simulink model "voima_7"  (R2022a)
settings: Solver=ode15s  StartTime=0.0  StopTime=1000  MaxStep=1  RelTol=1e-3  AbsTol=1e-3
values from neighbouring files (symbols this model uses):
  D = 1.2/a*0.5*tau    (= 37.7655389457)    [ex10.m]    (also in ex3.m = PID(3,i); ex4.m = 0; ex6.m = 37.77; ex7.m)
  fkul_0 = 35.7    [ex10.m]    (also in ex2.m; ex3.m; ex4.m; ex5.m)
  fp_0 = 35.7    [ex10.m]    (also in ex2.m; ex3.m; ex4.m; ex5.m)
  h1 = 8.3    [ex10.m]    (also in ex2.m; ex3.m; ex4.m; ex5.m)
  h2 = 21.0    (= 21)    [ex10.m]    (also in ex2.m; ex3.m; ex4.m; ex5.m)
  I = (1.2/a)/(2*tau)    (= 0.147521636507)    [ex10.m]    (also in ex3.m = PID(2,i); ex6.m = 0.1; ex7.m; ex8.m)
  k0 = 1.0    (= 1)    [ex10.m]    (also in ex2.m; ex3.m; ex4.m; ex5.m)
  k1 = 2.0    (= 2)    [ex10.m]    (also in ex2.m; ex3.m; ex4.m; ex5.m)
  k2 = 1/30    (= 0.0333333333333)    [ex10.m]    (also in ex2.m; ex3.m; ex4.m; ex5.m)
  k3 = 0.4    [ex10.m]    (also in ex2.m; ex3.m; ex4.m; ex5.m)
  k4 = 1/300    (= 0.00333333333333)    [ex10.m]    (also in ex2.m; ex3.m; ex4.m; ex5.m)
  k5 = 0.6    [ex10.m]    (also in ex2.m; ex3.m; ex4.m; ex5.m)
  k6 = 0.6    [ex10.m]    (also in ex2.m; ex3.m; ex4.m; ex5.m)
  k_in = k_in*15    (= 382.5)    [ex10.m]    (also in ex2.m = 25.5; ex3.m = 25.5; ex4.m = 25.5; ex5.m = 25.5)
  k_out = k_out*15    (= 3150)    [ex10.m]    (also in ex2.m = 210; ex3.m = 210; ex4.m = 210; ex5.m = 210)
  ma_0 = 150000.0    (= 150000)    [ex10.m]    (also in ex2.m; ex3.m; ex4.m; ex5.m)
  P = 1.2/a    (= 4.72069236821)    [ex10.m]    (also in ex3.m = PID(1,i); ex6.m = 5.66; ex7.m; ex8.m)
  pa_0 = 10.0    (= 10)    [ex10.m]    (also in ex2.m; ex3.m; ex4.m; ex5.m)
  pcp = 13.0    (= 13)    [ex10.m]    (also in ex2.m; ex3.m; ex4.m; ex5.m)
  pk_0 = 91.0    (= 91)    [ex10.m]    (also in ex2.m; ex3.m; ex4.m; ex5.m)
  pkp_0 = 89.25    [ex10.m]    (also in ex2.m; ex3.m; ex4.m; ex5.m)
  pvp_0 = 3.0    (= 3)    [ex10.m]    (also in ex2.m; ex3.m; ex4.m; ex5.m)
  T1 = 30.0    (= 30)    [ex10.m]    (also in ex2.m; ex3.m; ex4.m; ex5.m)
  Ts = 15.0    (= 15)    [ex10.m]    (also in ex2.m; ex3.m; ex4.m; ex5.m)
libraries: slpidlib x1
settings Model: Creator=meharju1  LastModifiedBy=Chris
settings SolverCC: AutoScaleAbsTol=off  AlgebraicLoopSolver=TrustRegion
settings DataIOCC: SaveFormat=Array  SignalLoggingSaveFormat=ModelDataLogs  SaveOutput=off  TimeSaveName=t
settings OptimizationCC: DefaultParameterBehavior=Inlined  InlineInvariantSignals=on  ExpressionDepthLimit=2147483647  EfficientFloat2IntCast=on  LifeSpan=inf
settings DebuggingCC: SaveWithParameterizedLinksMsg=none  MultiTaskCondExecSysMsg=none  UnconnectedInputMsg=warning  UnconnectedOutputMsg=warning  UnconnectedLineMsg=warning  UniqueDataStoreMsg=error  StateNameClashWarn=warning  PregeneratedLibrarySubsystemCodeDiagnostic=none  StrictBusMsg=ErrorOnBusTreatedAsVector  SFUnexpectedBacktrackingDiag=warning  SFNoUnconditionalDefaultTransitionDiag=warning  SFExecutionAtInitializationDiag=none  SFMachineParentedDataDiag=warning  ArithmeticOperatorsInVariantConditions=warning
settings HardwareCC: ProdBitPerPointer=32  ProdBitPerSizeT=32  ProdBitPerPtrDiffT=32  ProdLargestAtomicFloat=None  ProdIntDivRoundTo=Undefined  ProdEndianess=Unspecified  ProdWordSize=32  ProdHWDeviceType=32-bit Generic  TargetUnknown=on
settings ModelReferenceCC: PropagateSignalLabelsOutOfModel=off
settings SFSimCC: SimUseLocalCustomCode=off  CustomCodeUndefinedFunction=UseInterfaceOnly
settings RTWCC: RTWUseLocalCustomCode=off
settings CodeAppCC: StateflowObjectComments=on
settings GRTTargetCC: TargetLangStandard=C89/C90 (ANSI)  CombineOutputUpdateFcns=off  GRTInterface=on
settings ConfigComp: CovMetricSettings=dw  CovSaveCumulativeToWorkspaceVar=on  CovSaveSingleToWorkspaceVar=on  CovExternalEMLEnable=off

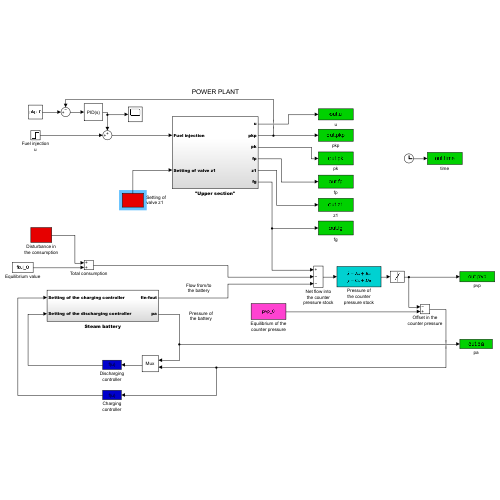
[thumbnail: Simulink's stored preview of the top-level diagram]
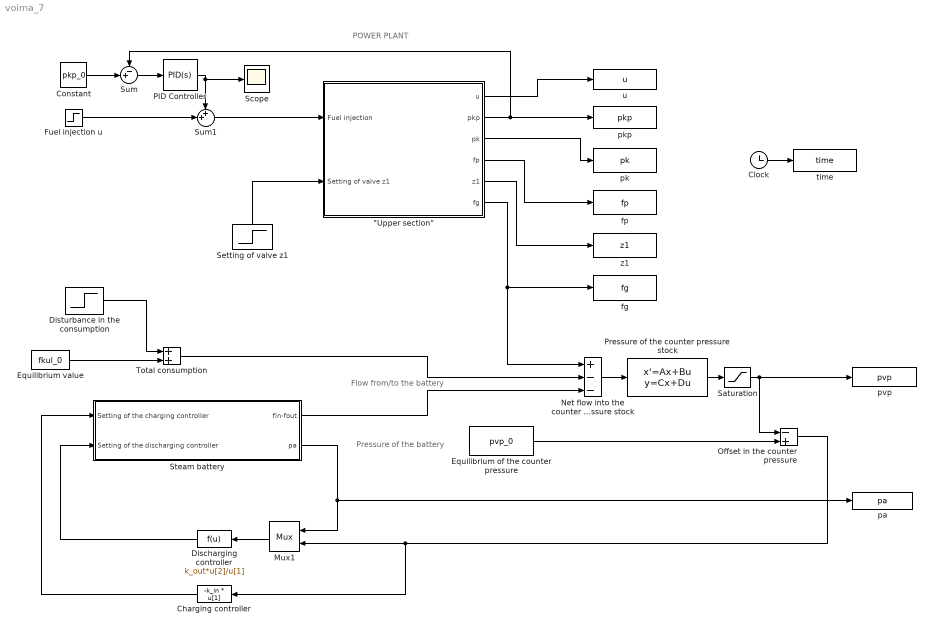
== system voima_7 ==
  note: POWER PLANT
  note: Flow from/to
      | the battery
  note: Pressure of
      | the battery
  "\"Upper section\"" : Subsystem
  Charging controller : Fcn  Expr=-k_in * u[1]
  Clock : Clock
  Constant : Constant  Value=pkp_0
  Discharging controller : Fcn  Expr=k_out*u[2]/u[1]
  Disturbance in the consumption : Step  Time=200  After=2  SampleTime=0
  Equilibrium of the counter pressure : Constant  Value=pvp_0
  Equilibrium value : Constant  Value=fkul_0
  Fuel injection u : Step  Time=200  Before=35.7  After=35.7  SampleTime=0
  Mux1 : Mux  Inputs=2
  Net flow into the counter pressure stock : Sum  Inputs=+--  InputSameDT=on  SaturateOnIntegerOverflow=on  OutDataTypeStr=Inherit: Same as first input
  Offset in the counter pressure : Sum  Inputs=-+  InputSameDT=on  SaturateOnIntegerOverflow=on  OutDataTypeStr=Inherit: Same as first input
  PID Controller : slpidlib/PID Controller  Controller=PID  Form=Parallel  TimeDomain=Continuous-time  UseExternalTs=off  SampleTime=-1  IntegratorMethod=Forward Euler  FilterMethod=Forward Euler  ControllerParametersSource=internal  P=P  I=I  UseKiTs=off  D=D  N=100  UseFilter=on  TunerSelectOption=Transfer Function Based (PID Tuner App)  InitialConditionSource=internal  InitialConditionForIntegrator=0  InitialConditionForFilter=0  DifferentiatorICPrevScaledInput=0  ExternalReset=none  TrackingMode=off  Kt=1  LimitOutput=off  SatLimitsSource=internal  UpperSaturationLimit=inf  LowerSaturationLimit=-inf  LinearizeAsGain=on  AntiWindupMode=none  Kb=1  POutMin=[]  POutMax=[]  IOutMin=[]  IOutMax=[]  DOutMin=[]  DOutMax=[]  NOutMin=[]  NOutMax=[]  SumOutMin=[]  SumOutMax=[]  SaturationOutMin=[]  SaturationOutMax=[]  PParamMin=[]  PParamMax=[]  IParamMin=[]  IParamMax=[]  DParamMin=[]  DParamMax=[]  NParamMin=[]  NParamMax=[]  KbParamMin=[]  KbParamMax=[]  KtParamMin=[]  KtParamMax=[]  KbOutMin=[]  KbOutMax=[]  KtOutMin=[]  KtOutMax=[]  IntegratorOutMin=[]  IntegratorOutMax=[]  FilterOutMin=[]  FilterOutMax=[]  SumI1OutMin=[]  SumI1OutMax=[]  SumI2OutMin=[]  SumI2OutMax=[]  SumI3OutMin=[]  SumI3OutMax=[]  SumI4OutMin=[]  SumI4OutMax=[]  SumDOutMin=[]  SumDOutMax=[]  DifferentiatorOutMin=[]  DifferentiatorOutMax=[]  FilterDiffOutCoefMin=[]  FilterDiffOutCoefMax=[]  ReciprocalOutMin=[]  ReciprocalOutMax=[]  SumDenOutMin=[]  SumDenOutMax=[]  SumNumOutMin=[]  SumNumOutMax=[]  DivideOutMin=[]  DivideOutMax=[]  UdiffTsProdOutMin=[]  UdiffTsProdOutMax=[]  NTsProdOutMin=[]  NTsProdOutMax=[]  UintegralTsProdOutMin=[]  UintegralTsProdOutMax=[]  UngainTsProdOutMin=[]  UngainTsProdOutMax=[]  IntegratorContinuousStateAttributes=''  IntegratorStateMustResolveToSignalObject=off  IntegratorRTWStateStorageClass=Auto  FilterContinuousStateAttributes=''  FilterStateMustResolveToSignalObject=off  FilterRTWStateStorageClass=Auto  ParallelPVariant=InternalParameters  IdealPVariant=Disabled  IVariant=InternalParameters  DVariant=InternalParameters  IntegratorVariant=Continuous  SatVariant=Disabled  AWVariant=Passthrough  PCopyVariant=Disabled  TRVariant=Disabled  FdbkBlocksVariant=Forward  IdealPFdbkVariant=Disabled  SatFdbkVariant=Disabled  DerivativeFilterVariant=ContFilter  NVariant=InternalParameters  NCopyVariant=Disabled  FilterICVariant=InternalICsFilter  IntegratorICVariant=InternalICs  ExternalResetVariant=Disabled  TRSumVariant=Passthrough  SumFdbkVariant=Disabled  SumVariant=Sum_PID  TsampFilterVariant=InternalTs  TsampNgainVariant=Passthrough  TsampIntegralVariant=Passthrough  ExternalSaturationOutDataTypeStr=Inherit: Same as second input  aMode=0
  Pressure of the counter pressure stock : StateSpace  A=0  B=k4  D=0  InitialCondition=pvp_0
  Saturation : Saturate  UpperLimit=100000  LowerLimit=0
  Scope : Scope
  Setting of valve z1 : Step  Time=200  Before=1  SampleTime=0
  Steam battery : Subsystem
  Sum : Sum  Inputs=-+|
  Sum1 : Sum  Inputs=++|
  Total consumption : Sum  InputSameDT=on  SaturateOnIntegerOverflow=on  OutDataTypeStr=Inherit: Same as first input
  fg : ToWorkspace  VariableName=fg
      settings: MaxDataPoints=2000
  fp : ToWorkspace  VariableName=fp
      settings: MaxDataPoints=2000
  pa : ToWorkspace  VariableName=pa
      settings: MaxDataPoints=2000
  pk : ToWorkspace  VariableName=pk
      settings: MaxDataPoints=2000
  pkp : ToWorkspace  VariableName=pkp
      settings: MaxDataPoints=2000
  pvp : ToWorkspace  VariableName=pvp
      settings: MaxDataPoints=2000
  time : ToWorkspace  VariableName=time
      settings: MaxDataPoints=2000
  u : ToWorkspace  VariableName=u
      settings: MaxDataPoints=2000
  z1 : ToWorkspace  VariableName=z1
      settings: MaxDataPoints=2000
  wires:
  Net flow into the counter pressure stock/1 -> Pressure of the counter pressure stock/1
  Equilibrium value/1 -> Total consumption/2
  Disturbance in the consumption/1 -> Total consumption/1
  Mux1/1 -> Discharging controller/1
  Equilibrium of the counter pressure/1 -> Offset in the counter pressure/2
  Steam battery/2(pa) -> pa/1, Mux1/1
  Total consumption/1 -> Net flow into the counter pressure stock/2
  Steam battery/1(fin-fout) -> Net flow into the counter pressure stock/3
  Discharging controller/1 -> Steam battery/2(Setting of the discharging controller)
  Offset in the counter pressure/1 -> Mux1/2, Charging controller/1
  "\"Upper section\""/1(u) -> u/1
  "\"Upper section\""/2(pkp) -> pkp/1, Sum/1
  "\"Upper section\""/3(pk) -> pk/1
  "\"Upper section\""/4(fp) -> fp/1
  Setting of valve z1/1 -> "\"Upper section\""/2(Setting of valve z1)
  Fuel injection u/1 -> Sum1/2
  Pressure of the counter pressure stock/1 -> Saturation/1
  Saturation/1 -> pvp/1, Offset in the counter pressure/1
  "\"Upper section\""/6(fg) -> Net flow into the counter pressure stock/1, fg/1
  "\"Upper section\""/5(z1) -> z1/1
  Charging controller/1 -> Steam battery/1(Setting of the charging controller)
  Clock/1 -> time/1
  Sum/1 -> PID Controller/1
  PID Controller/1 -> Scope/1, Sum1/1
  Constant/1 -> Sum/2
  Sum1/1 -> "\"Upper section\""/1(Fuel injection)

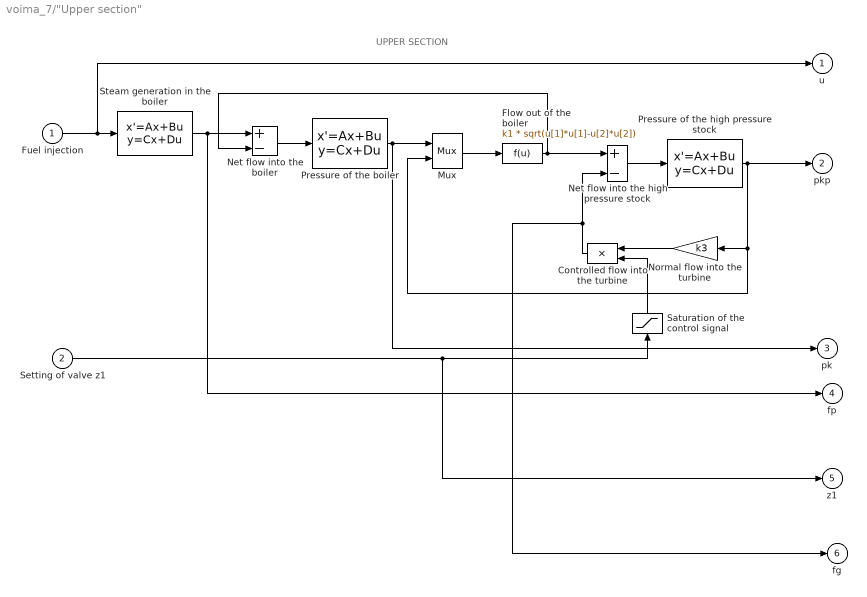
== system voima_7/"Upper section" ==
  note: UPPER SECTION
  Fuel injection : Inport
  Setting of valve z1 : Inport  Port=2
  Controlled flow into the turbine : Product  InputSameDT=on  RndMeth=Zero  SaturateOnIntegerOverflow=on  OutDataTypeStr=Inherit: Same as first input
  Flow out of the boiler : Fcn  Expr=k1 * sqrt(u[1]*u[1]-u[2]*u[2])
  Mux : Mux  Inputs=2
  Net flow into the boiler : Sum  Inputs=+-  InputSameDT=on  SaturateOnIntegerOverflow=on  OutDataTypeStr=Inherit: Same as first input
  Net flow into the high pressure stock : Sum  Inputs=+-  InputSameDT=on  SaturateOnIntegerOverflow=on  OutDataTypeStr=Inherit: Same as first input
  Normal flow into the turbine : Gain  Gain=k3  SaturateOnIntegerOverflow=on  OutDataTypeStr=Inherit: Same as input  ParamDataTypeStr=Inherit: Same as input
  Pressure of the boiler : StateSpace  A=0  B=1/Ts  D=0  InitialCondition=pk_0
  Pressure of the high pressure stock : StateSpace  A=0  B=k2  D=0  InitialCondition=pkp_0
  Saturation of the control signal : Saturate  UpperLimit=1.2  LowerLimit=0.8
  Steam generation in the boiler : StateSpace  A=-1/T1  B=k0 / T1  D=0  InitialCondition=fp_0
  u : Outport  VectorParamsAs1DForOutWhenUnconnected=off
  pkp : Outport  Port=2  VectorParamsAs1DForOutWhenUnconnected=off
  pk : Outport  Port=3  VectorParamsAs1DForOutWhenUnconnected=off
  fp : Outport  Port=4  VectorParamsAs1DForOutWhenUnconnected=off
  z1 : Outport  Port=5  VectorParamsAs1DForOutWhenUnconnected=off
  fg : Outport  Port=6  VectorParamsAs1DForOutWhenUnconnected=off
  wires:
  Saturation of the control signal/1 -> Controlled flow into the turbine/2
  Normal flow into the turbine/1 -> Controlled flow into the turbine/1
  Pressure of the high pressure stock/1 -> Normal flow into the turbine/1, Mux/2, pkp/1
  Net flow into the high pressure stock/1 -> Pressure of the high pressure stock/1
  Flow out of the boiler/1 -> Net flow into the boiler/2, Net flow into the high pressure stock/1
  Mux/1 -> Flow out of the boiler/1
  Net flow into the boiler/1 -> Pressure of the boiler/1
  Pressure of the boiler/1 -> Mux/1, pk/1
  Steam generation in the boiler/1 -> Net flow into the boiler/1, fp/1
  Controlled flow into the turbine/1 -> Net flow into the high pressure stock/2, fg/1
  Fuel injection/1 -> Steam generation in the boiler/1, u/1
  Setting of valve z1/1 -> Saturation of the control signal/1, z1/1

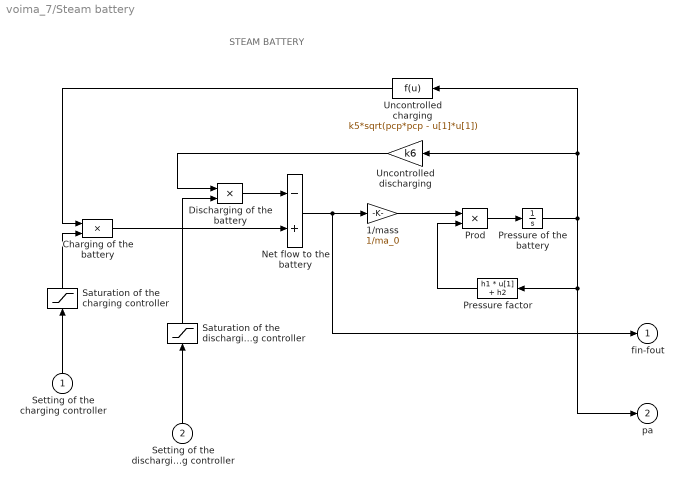
== system voima_7/Steam battery ==
  note: STEAM BATTERY
  Setting of the charging controller : Inport
  Setting of the discharging controller : Inport  Port=2
  1/mass : Gain  Gain=1/ma_0  SaturateOnIntegerOverflow=on  OutDataTypeStr=Inherit: Same as input  ParamDataTypeStr=Inherit: Same as input
  Charging of the battery : Product  InputSameDT=on  RndMeth=Zero  SaturateOnIntegerOverflow=on  OutDataTypeStr=Inherit: Same as first input
  Discharging of the battery : Product  InputSameDT=on  RndMeth=Zero  SaturateOnIntegerOverflow=on  OutDataTypeStr=Inherit: Same as first input
  Net flow to the battery : Sum  Inputs=-+  InputSameDT=on  SaturateOnIntegerOverflow=on  OutDataTypeStr=Inherit: Same as first input
  Pressure factor : Fcn  Expr="h1 * u[1]  + h2"
  Pressure of the battery : Integrator  InitialCondition=pa_0
  Prod : Product  InputSameDT=on  RndMeth=Zero  SaturateOnIntegerOverflow=on  OutDataTypeStr=Inherit: Same as first input
  Saturation of the charging controller : Saturate  UpperLimit=0  LowerLimit=0
  Saturation of the discharging controller : Saturate  UpperLimit=0  LowerLimit=0
  Uncontrolled charging : Fcn  Expr=k5*sqrt(pcp*pcp - u[1]*u[1])
  Uncontrolled discharging : Gain  Gain=k6  SaturateOnIntegerOverflow=on  OutDataTypeStr=Inherit: Same as input  ParamDataTypeStr=Inherit: Same as input
  fin-fout : Outport  VectorParamsAs1DForOutWhenUnconnected=off
  pa : Outport  Port=2  VectorParamsAs1DForOutWhenUnconnected=off
  wires:
  Saturation of the charging controller/1 -> Charging of the battery/2
  Saturation of the discharging controller/1 -> Discharging of the battery/2
  Uncontrolled discharging/1 -> Discharging of the battery/1
  Charging of the battery/1 -> Net flow to the battery/2
  Uncontrolled charging/1 -> Charging of the battery/1
  1/mass/1 -> Prod/1
  Pressure factor/1 -> Prod/2
  Prod/1 -> Pressure of the battery/1
  Pressure of the battery/1 -> Pressure factor/1, pa/1, Uncontrolled charging/1, Uncontrolled discharging/1
  Setting of the discharging controller/1 -> Saturation of the discharging controller/1
  Setting of the charging controller/1 -> Saturation of the charging controller/1
  Net flow to the battery/1 -> fin-fout/1, 1/mass/1
  Discharging of the battery/1 -> Net flow to the battery/1
